simulink model "myqpsk_optimized"  (R2025a)
settings: Solver=VariableStepAuto  StartTime=0.0  StopTime=2e-8  RelTol=1e-3
undefined symbols (not defined in the file): carrier_freq, PSK, raw_sample_rate, sample_rate, symbol_rate, window_len
libraries: simulink x2, dspsigops x2, commdigbbndpm3 x2, commchan3 x1, commrflib2 x1, commsink2 x1, dspfdesign x1, commrandsrc3 x1, dspstat3 x1
settings Model: Creator=IWMAI  LastModifiedBy=IWMAI

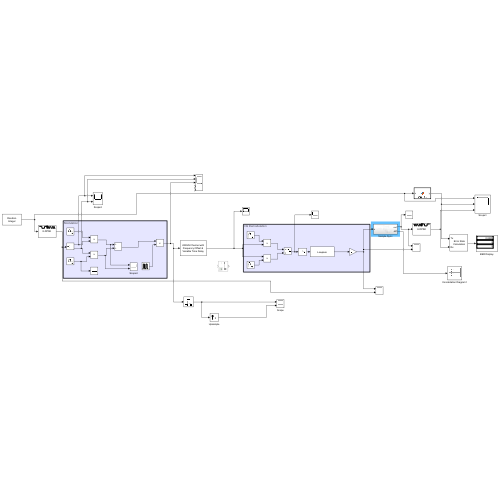
[thumbnail: Simulink's stored preview of the top-level diagram]
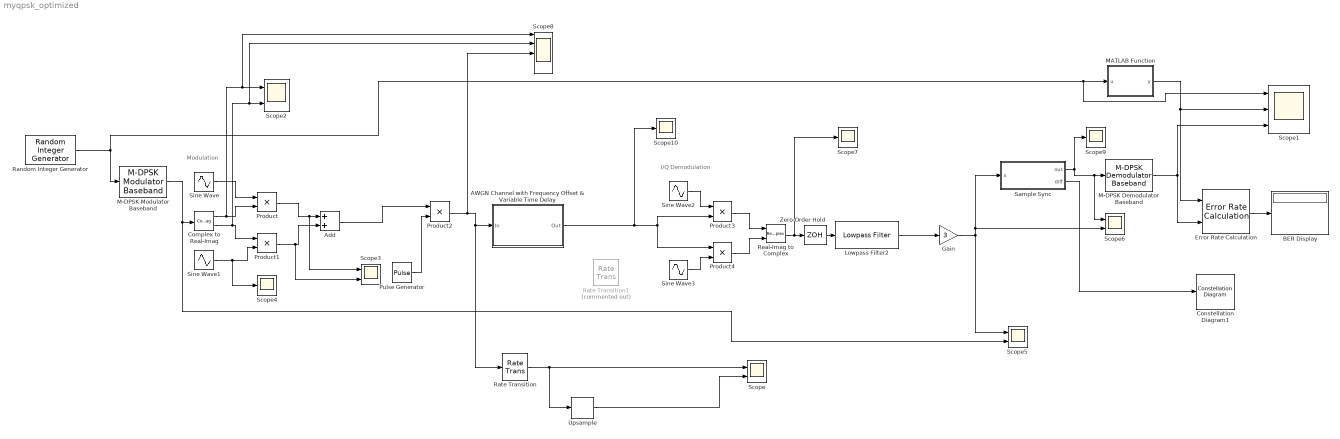
== system myqpsk_optimized ==
  note: Modulation
  note: I/Q Demodulation
  AWGN Channel with Frequency Offset & Variable Time Delay : Subsystem
      mask Display: disp('AWGN Channel with\nFrequency Offset & \nVariable Time Delay');
  Add : Sum
  BER Display : Display
  Complex to Real-Imag : ComplexToRealImag
  Constellation Diagram1 : ConstellationDiagram  WindowPosition=[564.000000,185.000000,600.000000,600.000000,]  Visible=on  ScopeFrameLocation=window  SymbolsToDisplaySource=Property  SymbolsToDisplay=1000  ReferenceConstellation=8-PSK  DefaultConfigurationName=comm.scopes.ConstellationDiagramBlockCfg
  Error Rate Calculation : commsink2/Error Rate Calculation  N=2  st_delay=0  cp_mode=Entire frame  subframe=qpsktxrx.BerMask  PMode=Port  WsName=ErrorVec  RsMode2=off  stop=off  numErr=100  maxBits=1e6
  Gain : Gain  Gain=3
  Lowpass Filter2 : dspfdesign/Lowpass Filter  FilterType=FIR  DesignForMinimumOrder=on  FilterOrder=50  PassbandFrequency=5e8  StopbandFrequency=1e9  PassbandRipple=0.1  StopbandAttenuation=80  SampleRateMode=Specify on dialog  SampleRate=sample_rate  SimulateUsing=Interpreted execution  roundingMode=Floor  coeffsDataTypeStr=fixdt(1,16)
  M-DPSK Demodulator Baseband : commdigbbndpm3/M-DPSK Demodulator Baseband  M=8  OutType=Integer  Dec=Gray  Ph=pi/4  outDtype1=Inherit via internal rule  outDtype2=Inherit via internal rule
  M-DPSK Modulator Baseband : commdigbbndpm3/M-DPSK Modulator Baseband  M=8  InType=Integer  Enc=Gray  Ph=pi/4  outDtype=double
  MATLAB Function : MATLAB Function  TreatAsAtomicUnit=on
  Product{,1..4} (5 alike) : Product
  Pulse Generator : DiscretePulseGenerator  PulseType=Time based  Period=2e-9  PulseWidth=37.5  PhaseDelay=480e-12  SampleTime=0.000001
  Random Integer Generator : commrandsrc3/Random Integer Generator  SetSize=8  SeedSource=Auto  Seed=0  SampleTime=2e-9  SamplesPerFrame=1  OutputDataType=double  SimulateUsing=Interpreted execution
  Rate Transition : RateTransition  OutPortSampleTime=1/raw_sample_rate
  Rate Transition1 : RateTransition  Commented=on  OutPortSampleTime=1/raw_sample_rate
  Real-Imag to Complex : RealImagToComplex
  Sample Sync : Subsystem
  Scope{,2..3,5..6} (5 alike) : Scope  NumInputPorts=2
      Scope settings: ActiveDisplayYMinimum=-0.97907888652158082  ActiveDisplayYMaximum=1.03084023747071
      Scope2 settings: ActiveDisplayYMinimum=-1  ActiveDisplayYMaximum=1  DataLoggingVariableName=ScopeData2
      Scope3 settings: ActiveDisplayYMinimum=-1.25  ActiveDisplayYMaximum=1.25  DataLoggingVariableName=ScopeData3
      Scope5 settings: ActiveDisplayYMinimum=-1  ActiveDisplayYMaximum=1  DataLoggingVariableName=ScopeData5
      Scope6 settings: ActiveDisplayYMinimum=-0.856702898817814  ActiveDisplayYMaximum=0.80553961271839547  DataLoggingVariableName=ScopeData6
  Scope1 : Scope  NumInputPorts=3
      settings: ActiveDisplayYMinimum=-0.87499999999999978  ActiveDisplayYMaximum=7.875
  Scope{4,7,9..10} (4 alike) : Scope
      Scope10 settings: ActiveDisplayYMinimum=-0.82041993362201715  ActiveDisplayYMaximum=0.81377093073528506  DataLoggingVariableName=ScopeData7
      Scope4 settings: ActiveDisplayYMinimum=-0.94006138687141994  ActiveDisplayYMaximum=1.1447903917408795  DataLoggingVariableName=ScopeData4
      Scope7 settings: ActiveDisplayYMinimum=-1  ActiveDisplayYMaximum=1  DataLoggingVariableName=ScopeData9
      Scope9 settings: ActiveDisplayYMinimum=-1  ActiveDisplayYMaximum=1  DataLoggingVariableName=ScopeData11
  Scope8 : Scope  NumInputPorts=5
      settings: ActiveDisplayYMinimum=-2.80770952361476  ActiveDisplayYMaximum=3.6963323752712358  DataLoggingVariableName=ScopeData8
  Sine Wave : Sin  Frequency=2*pi*4e9  Phase=pi/2  SampleTime=1/sample_rate
  Sine Wave1 : Sin  Frequency=2*pi*4e9  SampleTime=1/sample_rate
  Sine Wave2 : Sin  Frequency=2*pi*carrier_freq  Phase=pi/2  SampleTime=1 / sample_rate
  Sine Wave3 : Sin  Frequency=2*pi*carrier_freq  SampleTime=1 / sample_rate
  Upsample : dspsigops/Upsample  FactorSource=Dialog parameter  N=3  Nmax=16  phase=0  RateOptions=Allow multirate processing  ic=0  mode=Unused parameter value
      settings: LibrarySourceBlock=dsphdlsupportsigops/Upsample
  Zero-Order Hold : ZeroOrderHold  SampleTime=-1
  wires:
  Random Integer Generator/1 -> M-DPSK Modulator Baseband/1, MATLAB Function/1(u), Scope1/1
  M-DPSK Modulator Baseband/1 -> Scope5/2, Complex to Real-Imag/1
  Complex to Real-Imag/1 -> Scope8/1, Scope2/1, Product/2
  Sine Wave/1 -> Product/1
  Complex to Real-Imag/2 -> Scope8/2, Scope2/2, Product1/1
  Sine Wave1/1 -> Scope4/1, Product1/2
  Product/1 -> Scope3/1, Add/1
  Product1/1 -> Scope3/2, Add/2
  Add/1 -> Product2/1
  Pulse Generator/1 -> Product2/2
  Zero-Order Hold/1 -> Lowpass Filter2/1
  M-DPSK Demodulator Baseband/1 -> Scope1/3, Error Rate Calculation/2
  Sine Wave2/1 -> Product3/1
  Sine Wave3/1 -> Product4/2
  Gain/1 -> Scope5/1, Sample Sync/1(x), Scope6/2
  Sample Sync/1(out) -> M-DPSK Demodulator Baseband/1, Scope6/1, Scope9/1
  Product4/1 -> Real-Imag to Complex/2
  Product3/1 -> Real-Imag to Complex/1
  Real-Imag to Complex/1 -> Scope7/1, Zero-Order Hold/1
  Error Rate Calculation/1 -> BER Display/1
  MATLAB Function/1(y) -> Error Rate Calculation/1, Scope1/2
  Lowpass Filter2/1 -> Gain/1
  Sample Sync/2(diff) -> Constellation Diagram1/1
  Product2/1 -> Scope8/3, Rate Transition/1, AWGN Channel with Frequency Offset & Variable Time Delay/1(In)
  Rate Transition/1 -> Upsample/1, Scope/1
  Upsample/1 -> Scope/2
  AWGN Channel with Frequency Offset & Variable Time Delay/1(Out) -> Scope10/1, Product4/1, Product3/2

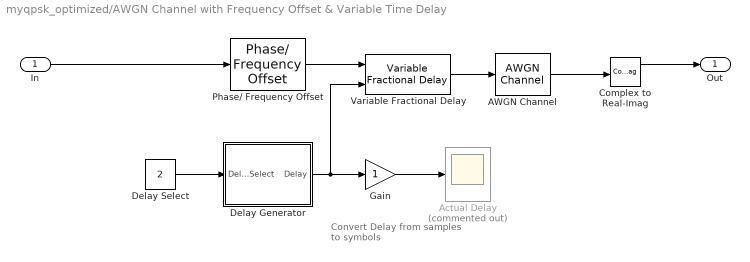
== system myqpsk_optimized/AWGN Channel with Frequency Offset & Variable Time Delay ==
  note: Convert Delay from
      | samples to symbols
  In : Inport
  AWGN Channel : commchan3/AWGN Channel  LegacyMode=off  NoiseMethod="Signal to noise ratio  (Eb/No)"  noiseMode="Signal to noise ratio  (Eb/No)"  EbNo=20  EsNo=15  SNR=15  BitsPerSymbol=2  SignalPower=0.5  SpecifySymbolPeriod=off  SamplesPerSymbol=2  SymbolPeriod=qpsktxrx.Tsym  VarianceSource=Parameter  Variance=1  RandomStream=mt19937ar with seed  Seed=2  SimulateUsing=Code generation
  Actual Delay : Scope  Commented=on
      settings: TimeSpan=0.1  TimeUnits=Metric (based on Time Span)  ActiveDisplayYMinimum=1.57813  ActiveDisplayYMaximum=2.04688  YLabel=Actual Delay (symbols)  DataLoggingVariableName=ScopeDataActualDelay
  Complex to Real-Imag : ComplexToRealImag
  Delay Generator : Subsystem
      mask Display: disp('Delay Generator')
  Delay Select : Constant  Value=2
  Gain : Gain
  Phase/ Frequency Offset : commrflib2/Phase// Frequency Offset  phaseOffset=47  freqPort=off  freqOffset=5000
  Variable Fractional Delay : dspsigops/Variable Fractional Delay  mode=OBSOLETE  modeActive=Linear  L=4  FarrowL=4  R=10  alpha=1  dmax=2266  InputProcessing=Columns as channels (frame based)  ic=0  noDFT=off  fallbackFIR=Clip to the minimum value necessary for centered kernel  fallbackFarrow=Clip to the minimum value necessary for centered kernel  roundingMode=Zero  overflowMode=off
  Out : Outport  VectorParamsAs1DForOutWhenUnconnected=off
  wires:
  Phase/ Frequency Offset/1 -> Variable Fractional Delay/1
  Variable Fractional Delay/1 -> AWGN Channel/1
  Delay Select/1 -> Delay Generator/1(Delay Select)
  Delay Generator/1(Delay) -> Variable Fractional Delay/2, Gain/1
  Gain/1 -> Actual Delay/1
  Complex to Real-Imag/1 -> Out/1
  In/1 -> Phase/ Frequency Offset/1
  AWGN Channel/1 -> Complex to Real-Imag/1

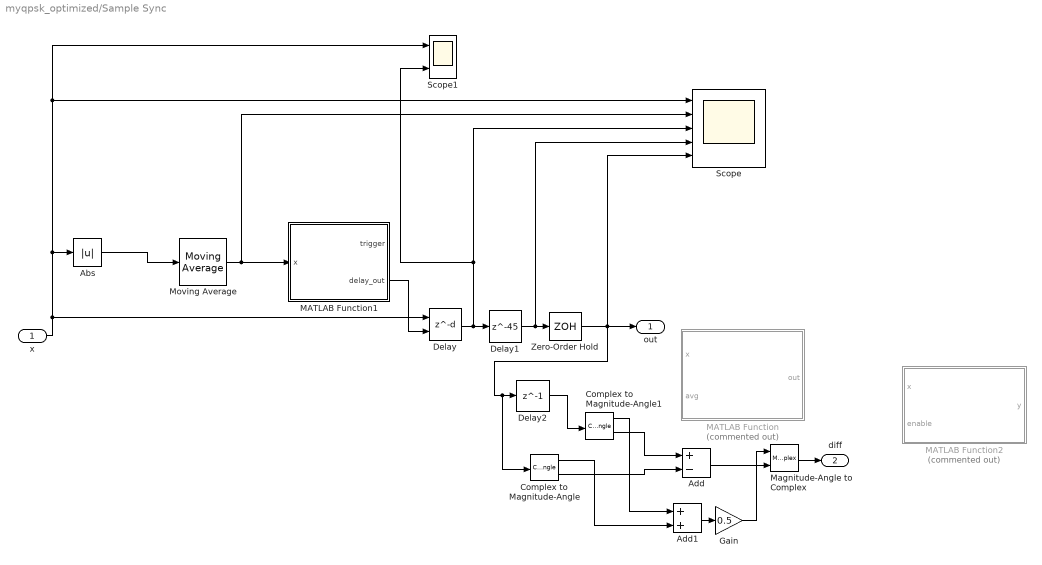
== system myqpsk_optimized/Sample Sync ==
  x : Inport
  Abs : Abs  SaturateOnIntegerOverflow=off
  Add : Sum  Inputs=+-
  Add1 : Sum
  Complex to Magnitude-Angle : ComplexToMagnitudeAngle
  Complex to Magnitude-Angle1 : ComplexToMagnitudeAngle
  Delay : Delay  DelayLengthSource=Input port  DelayLength=500  DelayLengthUpperLimit=3000
      settings: InputPortMap=u0,p1
  Delay1 : Delay  DelayLength=45
  Delay2 : Delay  DelayLength=1
  Gain : Gain  Gain=0.5
  MATLAB Function : MATLAB Function  Commented=on  TreatAsAtomicUnit=on
  MATLAB Function1 : MATLAB Function  TreatAsAtomicUnit=on
  MATLAB Function2 : MATLAB Function  Commented=on  TreatAsAtomicUnit=on
  Magnitude-Angle to Complex : MagnitudeAngleToComplex
  Moving Average : dspstat3/Moving Average  Method=Sliding window  ForgettingFactorPort=off  SpecifyWindowLength=on  WindowLength=window_len*6  OverlapLength=179  AllowArbitraryInputLength=off  ForgettingFactor=0.9  SimulateUsing=Interpreted execution
  Scope : Scope  NumInputPorts=5
      settings: ActiveDisplayYMinimum=-2.5553216850979239  ActiveDisplayYMaximum=2.608290111207836  DataLoggingVariableName=ScopeData7
  Scope1 : Scope  NumInputPorts=2
      settings: ActiveDisplayYMinimum=-1  ActiveDisplayYMaximum=1  DataLoggingVariableName=ScopeData10
  Zero-Order Hold : ZeroOrderHold  SampleTime=1/symbol_rate
  out : Outport
  diff : Outport  Port=2
  wires:
  x/1 -> Delay/1, Abs/1, Scope1/1, Scope/1
  Delay/1 -> Delay1/1, Scope/3, Scope1/2
  Abs/1 -> Moving Average/1
  Moving Average/1 -> MATLAB Function1/1(x), Scope/2
  Zero-Order Hold/1 -> Complex to Magnitude-Angle/1, Delay2/1, out/1, Scope/5
  MATLAB Function1/2(delay_out) -> Delay/2
  Delay1/1 -> Scope/4, Zero-Order Hold/1
  Delay2/1 -> Complex to Magnitude-Angle1/1
  Complex to Magnitude-Angle1/2 -> Add/1
  Complex to Magnitude-Angle/2 -> Add/2
  Add/1 -> Magnitude-Angle to Complex/2
  Magnitude-Angle to Complex/1 -> diff/1
  Complex to Magnitude-Angle1/1 -> Add1/1
  Complex to Magnitude-Angle/1 -> Add1/2
  Gain/1 -> Magnitude-Angle to Complex/1
  Add1/1 -> Gain/1

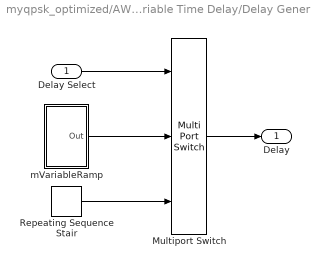
== system myqpsk_optimized/AWGN Channel with Frequency Offset & Variable Time Delay/Delay Generator ==
  Delay Select : Inport
  Multiport Switch : MultiPortSwitch  Inputs=2  OutDataTypeStr=double  SaturateOnIntegerOverflow=off  InputSameDT=off
  Repeating Sequence Stair : simulink/Sources/Repeating Sequence Stair  OutValues="[0       0.025        0.05       0.075         0.1       0.125        0.15       0.175         0.2       0.225        0.25       0.275         0.3       0.325        0.35       0.375         0.4       0.425        0.45       0.475         0.5       0.525        0.55       0.575         0.6       0.625        0.65       0.675         0.7       0.725        0.75       0.775         0.8       0.825        0.85       0.875         0.9       0.925        0.95       0.975           1       1.025        1.05       1.075         1.1       1.125        1.15       1.175         1.2       1.225        1.25       1.275         1.3       1.325        1.35       1.375         1.4       1.425        1.45       1.475         1.5       1.525        1.55       1.575         1.6       1.625        1.65       1.675         1.7       1.725        1.75       1.775         1.8       1.825        1.85       1.875         1.9       1.925        1.95       1.975           2       2.025        2.05       2.075         2.1       2.125        2.15       2.175         2.2       2.225        2.25       2.275         2.3       2.325        2.35       2.375         2.4       2.425        2.45       2.475         2.5       2.525        2.55       2.575         2.6       2.625        2.65       2.675         2.7       2.725        2.75       2.775         2.8       2.825        2.85       2.875         2.9       2.925        2.95       2.975           3       3.025        3.05       3.075         3.1       3.125        3.15       3.175         3.2       3.225        3.25       3.275         3.3       3.325        3.35       3.375         3.4       3.425        3.45       3.475         3.5       3.525        3.55       3.575         3.6       3.625        3.65       3.675         3.7       3.725        3.75       3.775         3.8       3.825        3.85       3.875         3.9       3.925        3.95       3.975           4       3.975        3.95       3.925         3.9       3.875        3.85       3.825         3.8       3.775        3.75       3.725         3.7       3.675        3.65       3.625         3.6       3.575        3.55       3.525         3.5       3.475        3.45       3.425         3.4       3.375        3.35       3.325         3.3       3.275        3.25       3.225         3.2       3.175        3.15       3.125         3.1       3.075        3.05       3.025           3       2.975        2.95       2.925         2.9       2.875        2.85       2.825         2.8       2.775        2.75       2.725         2.7       2.675        2.65       2.625         2.6       2.575        2.55       2.525         2.5       2.475        2.45       2.425         2.4       2.375        2.35       2.325         2.3       2.275        2.25       2.225         2.2       2.175        2.15       2.125         2.1       2.075        2.05       2.025           2       1.975        1.95       1.925         1.9       1.875        1.85       1.825         1.8       1.775        1.75       1.725         1.7       1.675        1.65       1.625         1.6       1.575        1.55       1.525         1.5       1.475        1.45       1.425         1.4       1.375        1.35       1.325         1.3       1.275        1.25       1.225         1.2       1.175        1.15       1.125         1.1       1.075        1.05       1.025           1       0.975        0.95       0.925         0.9       0.875        0.85       0.825         0.8       0.775        0.75       0.725         0.7       0.675        0.65       0.625         0.6       0.575        0.55       0.525         0.5       0.475        0.45       0.425         0.4       0.375        0.35       0.325         0.3       0.275        0.25       0.225         0.2       0.175        0.15       0.125         0.1       0.075        0.05       0.025]"  tsamp=0.02266  OutMin=[]  OutMax=[]  OutDataTypeStr=double  OutputDataTypeScalingMode=double  OutDataType=fixdt(0,8)  ConRadixGroup=Best Precision: Vector-wise  OutScaling=2^-12
  mVariableRamp : Subsystem
  Delay : Outport  VectorParamsAs1DForOutWhenUnconnected=off
  wires:
  Delay Select/1 -> Multiport Switch/1
  Repeating Sequence Stair/1 -> Multiport Switch/3
  mVariableRamp/1(Out) -> Multiport Switch/2
  Multiport Switch/1 -> Delay/1

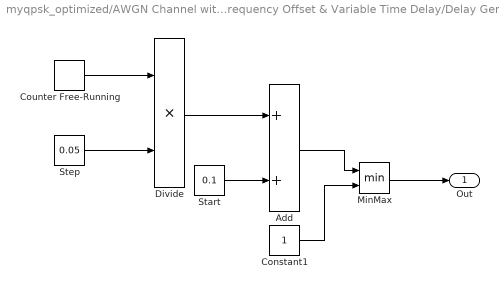
== system myqpsk_optimized/AWGN Channel with Frequency Offset & Variable Time Delay/Delay Generator/mVariableRamp ==
  Add : Sum
  Constant1 : Constant
  Counter Free-Running : simulink/Sources/Counter Free-Running  NumBits=64  tsamp=0.02266
  Divide : Product  Inputs=**
  MinMax : MinMax  Inputs=2
  Start : Constant  Value=0.1
  Step : Constant  Value=0.05
  Out : Outport  VectorParamsAs1DForOutWhenUnconnected=off
  wires:
  Counter Free-Running/1 -> Divide/1
  Step/1 -> Divide/2
  Divide/1 -> Add/1
  Start/1 -> Add/2
  Add/1 -> MinMax/1
  MinMax/1 -> Out/1
  Constant1/1 -> MinMax/2

== matlab function myqpsk_optimized/Sample Sync/MATLAB Function ==
  data: x input; out output; avg input
function out = peak_in_threshold_region(x, avg)
% x: 当前输入 sample（复数）
% avg: 当前 envelope sample（实数）
% out: 采样点（复数）

N = 3000;
TH = 0.8;

persistent x_buf avg_buf n_init

if isempty(x_buf)
    x_buf = complex(zeros(1, N));
    avg_buf = zeros(1, N);
    n_init = 0;
end

% Shift buffer
x_buf = [x_buf(2:end), x];
avg_buf = [avg_buf(2:end), avg];
n_init = n_init + 1;

out = complex(0, 0);

if n_init >= N
    % Step 1: 找最近一个连续满足 avg > 0.8 的区间
    region_mask = avg_buf > TH;

    % 从右往左找区域尾部（region_end）
    region_end = -1;
    for i = N:-1:1
        if region_mask(i)
            region_end = i;
            break;
        end
    end

    if region_end > 0
        % 往左找 region_start（区域起点）
        region_start = region_end;
        while region_start > 1 && region_mask(region_start - 1)
            region_start = region_start - 1;
        end

        % Step 2: 在这个区间内找最大值的位置
        [~, rel_idx] = max(avg_buf(region_start:region_end));
        abs_idx = region_start + rel_idx - 1;

        % Step 3: 输出对应的 x
        out = x_buf(max(1, abs_idx - 350));
        % disp(n_init + " " + abs_idx);
    end
end

== matlab function myqpsk_optimized/Sample Sync/MATLAB Function2 ==
  data: x input; y output; enable input
function y = enable_hold(x, enable)

N = 1000;
delay = 350;

persistent temp_y x_buf

if isempty(temp_y)
    temp_y = complex(x);
    x_buf = complex(zeros(1, N));
end

x_buf = [x_buf(2:end), x];

if enable
    temp_y = x_buf(N - delay);
end

y = temp_y;

== matlab function myqpsk_optimized/MATLAB Function ==
  data: u input; y output
function y = drop_1st(u)

persistent temp

y = u;

if isempty(temp)
    y = 0;
    temp = 0;
end

== matlab function myqpsk_optimized/Sample Sync/MATLAB Function1 ==
  data: x input; trigger output; delay_out output
function [trigger, delay_out] = peak_clock_with_cd(x)
% 输入:
%   x - 实时尖峰信号（实数或复数）
% 输出:
%   trigger - 是否触发采样
%   delay_out - 当前的采样 delay 值（用于 Variable Delay 控制）

N = 5;              % 滑动窗口长度
sample_rate = 4e10;
CD_LEN = int32(2e-9 * sample_rate * 0.8);      % Cooldown 冷却期
RESET_DELAY = int32(750e-12 * sample_rate / 2);  % 触发时 delay 初始值

persistent buf cd_counter delay

if isempty(buf)
    buf = complex(zeros(1, N));
    cd_counter = int32(0);
    delay = RESET_DELAY;  % 初始化 delay 为350
end

% 每次都更新缓冲区
buf = [buf(2:end), x];

% 默认输出
trigger = 0;
delay_out = delay;

% Cooldown 状态时 delay 仍然累加
if cd_counter > 0
    cd_counter = cd_counter - 1;
end

% 检测是否为局部 peak
if abs(buf(2)) < abs(buf(3)) && abs(buf(3)) > abs(buf(4)) && cd_counter == 0
    trigger = 1;
    cd_counter = CD_LEN;
    delay = RESET_DELAY;     % 💡 触发时 delay 重置为 350
else
    delay = delay + 1;       % 💡 否则每次递增
end

% 输出当前 delay
delay_out = delay;
